simulink model "mEnabSSVarSize_nestedvirtbuswbo"  (Simulink 8.0)
settings: Solver=FixedStepDiscrete  StartTime=0.0  StopTime=10.0  FixedStep=0.2  RelTol=1e-3
PreLoadFcn:
  | load mvardims_bus2.mat;
CloseFcn:
  | clear a b;
settings Model: FPTRunName=Active  Creator=djia  LastModifiedBy=mtocci  ExtModeAutoUpdateStatusClock=off
settings DataIOCC: SaveFormat=StructureWithTime  SignalLoggingSaveFormat=ModelDataLogs
settings OptimizationCC: InlineParams=on  InitFltsAndDblsToZero=on  EfficientMapNaN2IntZero=off
settings DebuggingCC: FcnCallInpInsideContextMsg=Use local settings
settings GRTTargetCC: TargetFcnLib=ansi_tfl_tmw.mat  CombineOutputUpdateFcns=off

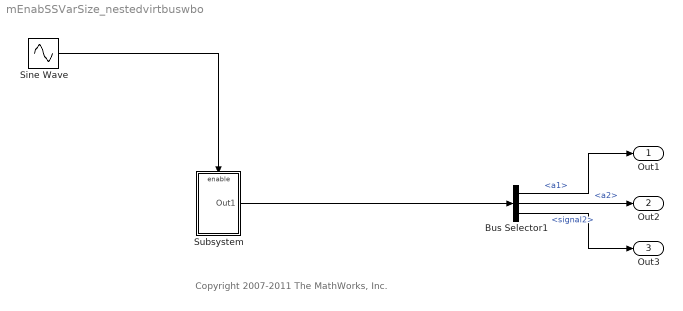
== system mEnabSSVarSize_nestedvirtbuswbo ==
  note: Copyright 2007-2011 The MathWorks, Inc.
  Bus Selector1 : BusSelector  OutputSignals=signal1.a1,signal1.a2,signal2
  Sine Wave : Sin  SampleTime=0.2
  Subsystem : Subsystem
  Out1 : Outport
  Out2 : Outport  Port=2
  Out3 : Outport  Port=3
  wires:
  Bus Selector1/1 -> Out1/1  "<a1>"
  Bus Selector1/2 -> Out2/1  "<a2>"
  Bus Selector1/3 -> Out3/1  "<signal2>"
  Subsystem/1(Out1) -> Bus Selector1/1
  Sine Wave/1 -> Subsystem/Enable

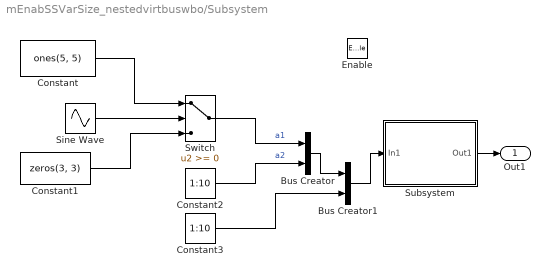
== system mEnabSSVarSize_nestedvirtbuswbo/Subsystem ==
  Enable : EnablePort  PropagateVarSize=During execution
  Bus Creator : BusCreator  Inputs=2  OutDataTypeStr=Bus: a
  Bus Creator1 : BusCreator  Inputs=2  OutDataTypeStr=Bus: b
  Constant : Constant  Value=ones(5, 5)
  Constant1 : Constant  Value=zeros(3, 3)
  Constant2 : Constant  Value=1:10  SampleTime=0.2
  Constant3 : Constant  Value=1:10  SampleTime=0.2
  Sine Wave : Sin  SampleTime=0.2
  Subsystem : Subsystem  TreatAsAtomicUnit=on
  Switch : Switch  AllowDiffInputSizes=on
  Out1 : Outport  InitialOutput=0
  wires:
  Switch/1 -> Bus Creator/1  "a1"
  Constant/1 -> Switch/1
  Constant2/1 -> Bus Creator/2  "a2"
  Sine Wave/1 -> Switch/2
  Constant1/1 -> Switch/3
  Bus Creator/1 -> Bus Creator1/1
  Constant3/1 -> Bus Creator1/2
  Bus Creator1/1 -> Subsystem/1(In1)
  Subsystem/1(Out1) -> Out1/1

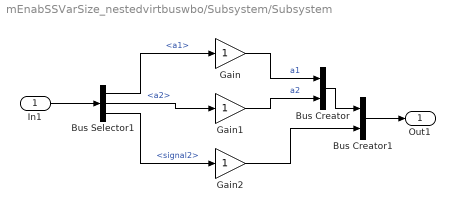
== system mEnabSSVarSize_nestedvirtbuswbo/Subsystem/Subsystem ==
  In1 : Inport
  Bus Creator : BusCreator  Inputs=2  OutDataTypeStr=Bus: a
  Bus Creator1 : BusCreator  Inputs=2  OutDataTypeStr=Bus: b
  Bus Selector1 : BusSelector  OutputSignals=signal1.a1,signal1.a2,signal2
  Gain : Gain
  Gain1 : Gain
  Gain2 : Gain
  Out1 : Outport
  wires:
  Bus Selector1/1 -> Gain/1  "<a1>"
  Bus Selector1/2 -> Gain1/1  "<a2>"
  Gain/1 -> Bus Creator/1  "a1"
  Gain1/1 -> Bus Creator/2  "a2"
  Bus Creator/1 -> Bus Creator1/1
  Gain2/1 -> Bus Creator1/2
  Bus Creator1/1 -> Out1/1
  In1/1 -> Bus Selector1/1
  Bus Selector1/3 -> Gain2/1  "<signal2>"
